simulink model "NonLinear_IPend_PP_Michigan_MSAM"  (Simulink 7.9)
settings: Solver=ode45  StartTime=0.0  StopTime=time_span  RelTol=1e-3
values from neighbouring files (symbols this model uses):
  outstr = sim_model    [RunCtrlModel.m]    (also in RunPertModels_sym.m = GetEqnStr_sym(model_eqns(j),p.allvars,'eqn'))
  samp_time = p.simulation.samp_time    [RunCtrlModel.m]    (also in RunPertModels_sym.m)
undefined symbols (not defined in the file or in its folder): p
libraries: dspsrcs4 x1
settings Model: Creator=Kushal  LastModifiedBy=Kourosh Danai
settings SolverCC: ZeroCrossAlgorithm=Adaptive  AlgebraicLoopSolver=LineSearch
settings DebuggingCC: SignalRangeChecking=error  AlgebraicLoopMsg=none
settings GRTTargetCC: CombineOutputUpdateFcns=off  GRTInterface=on

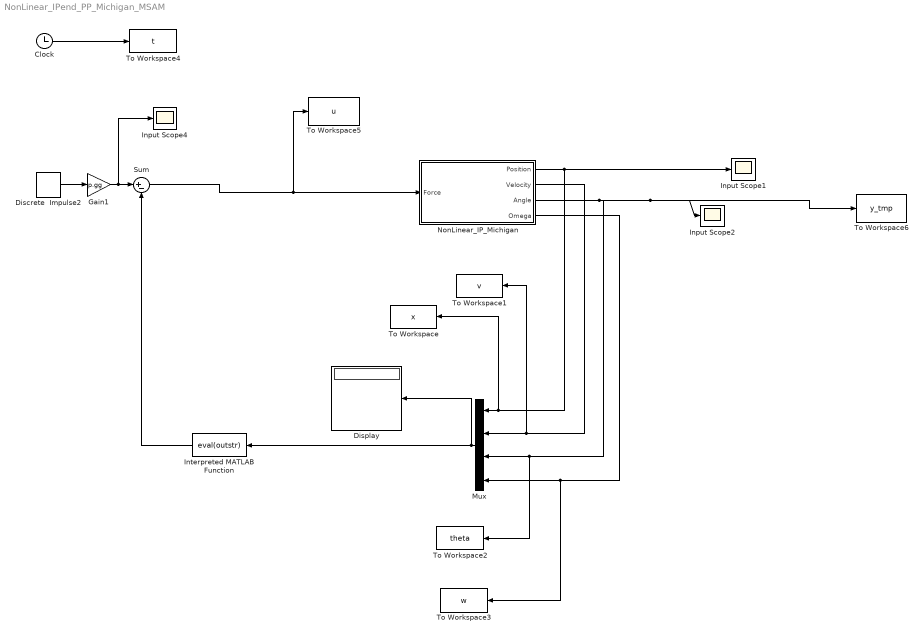
== system NonLinear_IPend_PP_Michigan_MSAM ==
  Clock : Clock
  Discrete  Impulse2 : dspsrcs4/Discrete  Impulse  Delay=0  SampleTime=1  FrameSample=1  dataType=double  isSigned=on  wordLen=16  udDataType=sfix(16)  fracBitsMode=Best precision  numFracBits=15  OutDataTypeStr=double  LastOutDataTypeStr=double
  Display : Display
  Gain1 : Gain  Gain=p.gg
  Input Scope1 : Scope
      settings: YMin=2.3e+007  YMax=2.8e+007
  Input Scope2 : Scope
  Input Scope4 : Scope
      settings: SaveName=ScopeData3
  Interpreted MATLAB Function : MATLABFcn  MATLABFcn=eval(outstr)
  Mux : Mux
  NonLinear_IP_Michigan : Subsystem
  Sum : Sum  Inputs=|+-
  To Workspace : ToWorkspace  VariableName=x  SampleTime=samp_time  SaveFormat=Structure
  To Workspace1 : ToWorkspace  VariableName=v  SampleTime=samp_time  SaveFormat=Structure
  To Workspace2 : ToWorkspace  VariableName=theta  SampleTime=samp_time  SaveFormat=Structure
  To Workspace3 : ToWorkspace  VariableName=w  SampleTime=samp_time  SaveFormat=Structure
  To Workspace4 : ToWorkspace  VariableName=t  SampleTime=samp_time
  To Workspace5 : ToWorkspace  VariableName=u  SampleTime=samp_time
  To Workspace6 : ToWorkspace  VariableName=y_tmp  SampleTime=samp_time
  wires:
  NonLinear_IP_Michigan/1(Position) -> Input Scope1/1, Mux/1, To Workspace/1
  NonLinear_IP_Michigan/3(Angle) -> Mux/3, To Workspace2/1, Input Scope2/1, To Workspace6/1
  NonLinear_IP_Michigan/4(Omega) -> Mux/4, To Workspace3/1
  Mux/1 -> Display/1, Interpreted MATLAB Function/1
  NonLinear_IP_Michigan/2(Velocity) -> Mux/2, To Workspace1/1
  Clock/1 -> To Workspace4/1
  Interpreted MATLAB Function/1 -> Sum/2
  Discrete  Impulse2/1 -> Gain1/1
  Sum/1 -> NonLinear_IP_Michigan/1(Force), To Workspace5/1
  Gain1/1 -> Sum/1, Input Scope4/1

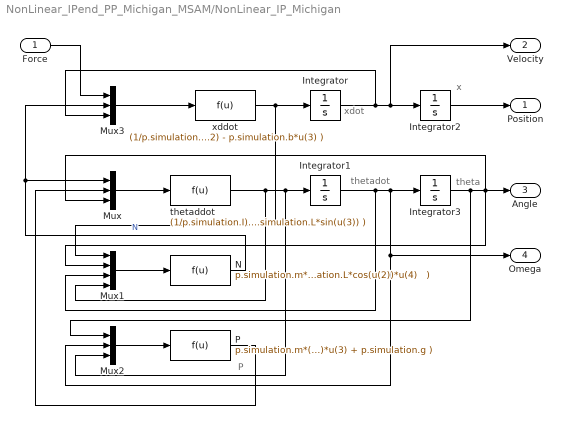
== system NonLinear_IPend_PP_Michigan_MSAM/NonLinear_IP_Michigan ==
  note: xdot
  note: x
  note: thetadot
  note: theta
  note: P
  Force : Inport
  Integrator : Integrator  ContinuousStateAttributes='xdot'
  Integrator1 : Integrator  ContinuousStateAttributes='thetadot'
  Integrator2 : Integrator  ContinuousStateAttributes='x'
  Integrator3 : Integrator  ContinuousStateAttributes='theta'
  Mux : Mux  Inputs=3
  Mux1 : Mux
  Mux2 : Mux  Inputs=3
  Mux3 : Mux  Inputs=3
  N : Fcn  Expr="p.simulation.m*( u(1) + p.simulation.L * sin(u(2))* (u(3)^2)  - p.simulation.L*cos(u(2))*u(4)   )"
  P : Fcn  Expr=p.simulation.m*(-p.simulation.L*cos(u(1))*(u(2)^2) - p.simulation.L*sin(u(1))*u(3) + p.simulation.g )
  thetaddot : Fcn  Expr=(1/p.simulation.I)*( u(1)*p.simulation.L*cos(u(3)) + u(2)*p.simulation.L*sin(u(3)) )
  xddot : Fcn  Expr=(1/p.simulation.M)*( u(1) - u(2) - p.simulation.b*u(3) )
  Position : Outport  OutMin=-100  OutMax=+100
  Velocity : Outport  Port=2
  Angle : Outport  Port=3
  Omega : Outport  Port=4
  wires:
  Integrator/1 -> Mux3/3, Integrator2/1, Velocity/1
  Integrator1/1 -> Mux1/3, Integrator3/1, Mux2/2, Omega/1
  xddot/1 -> Integrator/1, Mux1/1
  thetaddot/1 -> Mux1/4, Integrator1/1, Mux2/3
  Mux/1 -> thetaddot/1
  Integrator2/1 -> Position/1
  Integrator3/1 -> Angle/1, Mux1/2, Mux/3, Mux2/1
  Mux1/1 -> N/1
  Mux3/1 -> xddot/1
  Force/1 -> Mux3/1
  N/1 -> Mux3/2, Mux/1  "N"
  Mux2/1 -> P/1
  P/1 -> Mux/2
